simulink model "Power_Electronics_Simulation"  (R2017a)
settings: Solver=VariableStepAuto  StartTime=0.0  StopTime=3.5  MaxStep=1e-4  RelTol=1e-3
libraries: powerlib x15, simulink x1
settings Model: Creator=Shashank Sharma  LastModifiedBy=Shashank Sharma

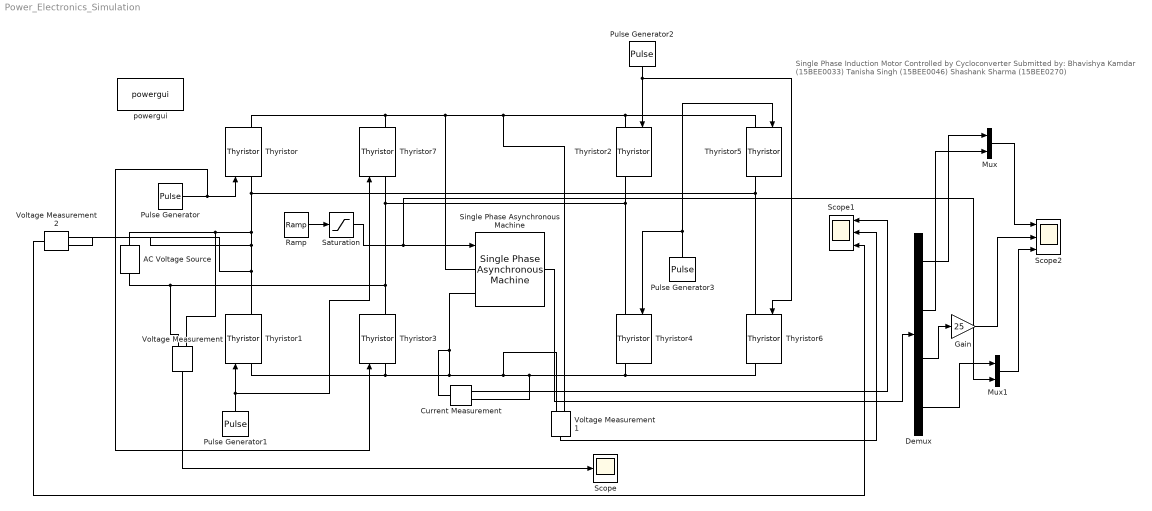
== system Power_Electronics_Simulation ==
  note: Single Phase Induction Motor Controlled by Cycloconverter
      | Submitted by:
      | Bhavishya Kamdar (15BEE0033)
      | Tanisha Singh (15BEE0046)
      | Shashank Sharma (15BEE0270)
  AC Voltage Source : powerlib/Electrical Sources/AC Voltage Source  Amplitude=250  Phase=0  Frequency=50  SampleTime=0  Measurements=None  BusType=swing  Pref=10e3  Qref=0  Qmin=-inf  Qmax=+inf
  Current Measurement : powerlib/Measurements/Current Measurement  PhasorSimulation=off  OutputType=Complex  PSBequivalent=0
  Demux : Demux
  Gain : Gain  Gain=25
  Mux : Mux  Inputs=2
  Mux1 : Mux  Inputs=2
  Pulse Generator : DiscretePulseGenerator  PulseType=Time based  Period=40e-3  PulseWidth=50
  Pulse Generator1 : DiscretePulseGenerator  PulseType=Time based  Period=40e-3  PulseWidth=50  PhaseDelay=10e-3
  Pulse Generator2 : DiscretePulseGenerator  PulseType=Time based  Period=40e-3  PulseWidth=50  PhaseDelay=20e-3
  Pulse Generator3 : DiscretePulseGenerator  PulseType=Time based  Period=40e-3  PulseWidth=50  PhaseDelay=30e-3
  Ramp : simulink/Sources/Ramp  slope=1  start=0  X0=0
  Saturation : Saturate
  Scope : Scope
  Scope1 : Scope  NumInputPorts=3
  Scope2 : Scope  NumInputPorts=3
  Single Phase Asynchronous Machine : powerlib/Machines/Single Phase Asynchronous Machine  MechanicalLoad=Torque Tm  UNITS=SI  MachineType=Split Phase  MeasurementBus=off  NominalParameters="[ .25*746  110  60]"  MainWindingStator="[2.02  7.4e-3]"  MainWindingRotor="[4.12  5.6e-3]"  MutualInductance=0.1772  AuxiliaryWinding="[7.14  8.5e-3]"  Mechanical="[0.0146  0  2 1.18]"  CapacitorStart="[2  254.7e-6]"  CapacitorRun="[18  21.1e-6]"  DisconnectionSpeed=75  InitialSpeed=0  DataType=SI  TsPowergui=0  TsBlock=-1
      settings: SourceProductName=Simscape Power Systems  SourceProductBaseCode=PS
  Thyristor{,1..7} (8 alike) : powerlib/Power Electronics/Thyristor  Ron=0.001  Lon=0  Vf=0.8  IC=0  Rs=500  Cs=250e-9  Measurements=on
  Voltage Measurement : powerlib/Measurements/Voltage Measurement  PhasorSimulation=off  OutputType=Complex  PSBequivalent=0
  Voltage Measurement1 : powerlib/Measurements/Voltage Measurement  PhasorSimulation=off  OutputType=Complex  PSBequivalent=0
  Voltage Measurement2 : powerlib/Measurements/Voltage Measurement  PhasorSimulation=off  OutputType=Complex  PSBequivalent=0
  powergui : powerlib/powergui  Priority=1  SimulationMode=Continuous  SampleTime=50e-6  frequency=60  Iterations=50  frequencyindice=50  Pbase=100e6  ErrMax=1e-4  UnitsV=kV  UnitsW=MW  buscounter=0  FunctionMessages=off  echomessages=off  EnableUseOfTLC=off  CurrentSourceSwitches=off  DisableSnubberDevices=off  DisableRonSwitches=off  DisableVfSwitches=off  DisplayEquations=off  SolverType=Tustin/Backward Euler (TBE)  Interpol=off  ExternalGateDelay=off  methode=off  Ts=100  x0status=blocks  SPID=on  SwTol=0  HookPort=off  RestoreLinks=warning  ResistiveCurrentMeasurement=off  Frange=[0:2:500]  Ylog=off  Xlog=on  ShowGrid=off  save=off  variable=ZData  structure=0  ZoomFFT=off  StartTime=0.0  cycles=1  DisplayStyle=1  fundamental=60  FreqAxis=off  MaxFrequency=1000  frequencyindicesteady=1  RmsSteady=1  display=off
  wires:
  Pulse Generator1/1 -> Thyristor7/1, Thyristor1/1
  Pulse Generator2/1 -> Thyristor6/1, Thyristor2/1
  Pulse Generator/1 -> Thyristor/1, Thyristor3/1
  Voltage Measurement/1 -> Scope/1
  Pulse Generator3/1 -> Thyristor5/1, Thyristor4/1
  Voltage Measurement2/1 -> Scope1/3
  Ramp/1 -> Saturation/1
  Saturation/1 -> Mux1/2, Single Phase Asynchronous Machine/1
  Voltage Measurement1/1 -> Scope1/2
  Current Measurement/1 -> Scope1/1
  Single Phase Asynchronous Machine/1 -> Demux/1
  Demux/4 -> Mux1/1
  Demux/1 -> Mux/1
  Demux/2 -> Mux/2
  Mux1/1 -> Scope2/3
  Demux/3 -> Gain/1
  Mux/1 -> Scope2/1
  Gain/1 -> Scope2/2
  connections:
  AC Voltage Source/LConn1 -- Thyristor3/RConn1 -- Thyristor4/LConn1 -- Thyristor2/RConn1 -- Thyristor7/LConn1 -- Voltage Measurement/LConn2
  Thyristor2/LConn1 -- Thyristor5/LConn1 -- Voltage Measurement1/LConn1 -- Single Phase Asynchronous Machine/LConn1 -- Thyristor/RConn1 -- Thyristor7/RConn1
  Thyristor3/LConn1 -- Current Measurement/LConn1 -- Single Phase Asynchronous Machine/LConn2 -- Current Measurement/RConn1 -- Thyristor6/RConn1 -- Thyristor4/RConn1 -- Voltage Measurement1/LConn2 -- Thyristor1/LConn1
  Thyristor6/LConn1 -- Voltage Measurement2/LConn2 -- Thyristor1/RConn1 -- Voltage Measurement2/LConn1 -- AC Voltage Source/RConn1 -- Voltage Measurement/LConn1 -- Thyristor/LConn1 -- Thyristor5/RConn1
